simulink model "practica5_simulink"  (R2024a)
settings: Solver=ode4  StartTime=0.0  StopTime=0.5  FixedStep=0.000001  RelTol=1e-3
values from neighbouring files (symbols this model uses):
  den = [1, R/L, 1/(L*C)]    [pr5pt1.m]
  Kd = 0.01    [pr5pt1.m]
  Ki = 1000    [pr5pt1.m]
  Kp = 10    [pr5pt1.m]
  num = [1/(L*C)]    [pr5pt1.m]
libraries: slpidlib x3
settings Model: Creator=Monsty  LastModifiedBy=Monsty

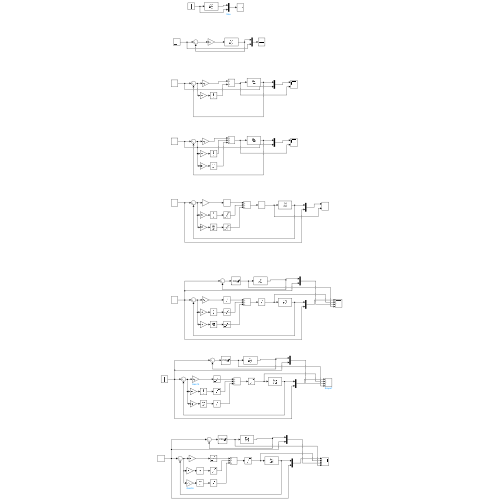
[thumbnail: Simulink's stored preview of the top-level diagram]
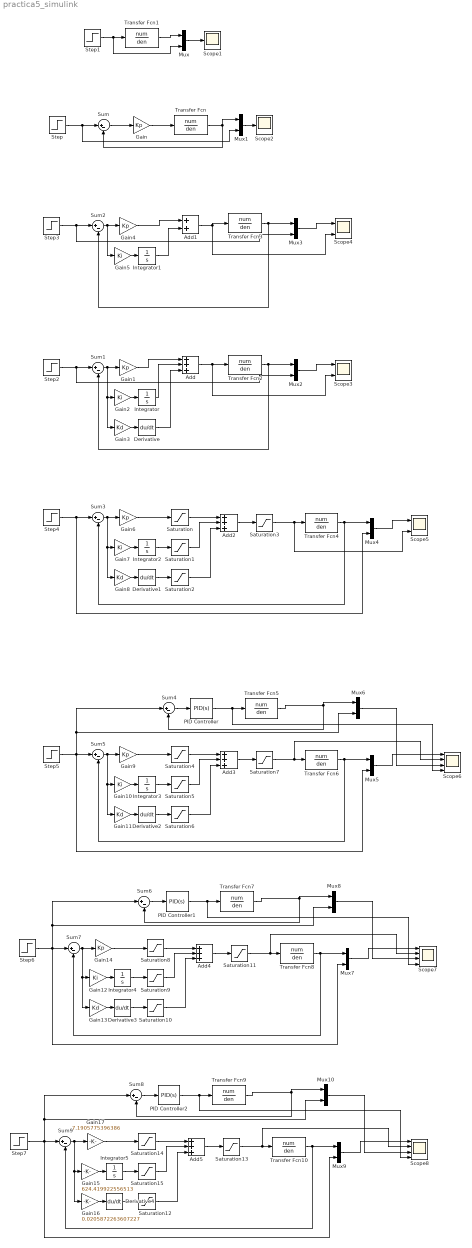
== system practica5_simulink ==
  Add{,2..5} (5 alike) : Sum  Inputs=+++
  Add1 : Sum
  Derivative{,1..4} (5 alike) : Derivative
  Gain{,1,4,6,9,14} (6 alike) : Gain  Gain=Kp
  Gain{2,5,7,10,12} (5 alike) : Gain  Gain=Ki
  Gain{3,8,11,13} (4 alike) : Gain  Gain=Kd
  Gain15 : Gain  Gain=624.419922556513
  Gain16 : Gain  Gain=0.0205872263607227
  Gain17 : Gain  Gain=7.1905775396386
  Integrator{,1..5} (6 alike) : Integrator
  Mux{,1..10} (11 alike) : Mux  Inputs=2
  PID Controller : slpidlib/PID Controller  Controller=PID  Form=Parallel  TimeDomain=Continuous-time  UseExternalTs=off  SampleTime=-1  IntegratorMethod=Forward Euler  FilterMethod=Forward Euler  ControllerParametersSource=internal  P=10  I=100  UseKiTs=off  D=0.01  UseExternalDerivativeSource=off  N=1000000  UseFilter=on  TunerSelectOption=Transfer Function Based (PID Tuner App)  InitialConditionSource=internal  InitialConditionForIntegrator=0  InitialConditionForFilter=0  DifferentiatorICPrevScaledInput=0  ExternalReset=none  TrackingMode=off  Kt=1  LimitOutput=on  SatLimitsSource=internal  UpperSaturationLimit=15  LowerSaturationLimit=-15  LinearizeAsGain=on  AntiWindupMode=none  Kb=1  LimitIntegrator=off  UpperIntegratorSaturationLimit=inf  LowerIntegratorSaturationLimit=-inf  POutMin=[]  POutMax=[]  IOutMin=[]  IOutMax=[]  DOutMin=[]  DOutMax=[]  NOutMin=[]  NOutMax=[]  SumOutMin=[]  SumOutMax=[]  SaturationOutMin=[]  SaturationOutMax=[]  PParamMin=[]  PParamMax=[]  IParamMin=[]  IParamMax=[]  DParamMin=[]  DParamMax=[]  NParamMin=[]  NParamMax=[]  KbParamMin=[]  KbParamMax=[]  KtParamMin=[]  KtParamMax=[]  KbOutMin=[]  KbOutMax=[]  KtOutMin=[]  KtOutMax=[]  IntegratorOutMin=[]  IntegratorOutMax=[]  FilterOutMin=[]  FilterOutMax=[]  SumI1OutMin=[]  SumI1OutMax=[]  SumI2OutMin=[]  SumI2OutMax=[]  SumI3OutMin=[]  SumI3OutMax=[]  SumI4OutMin=[]  SumI4OutMax=[]  SumDOutMin=[]  SumDOutMax=[]  DifferentiatorOutMin=[]  DifferentiatorOutMax=[]  FilterDiffOutCoefMin=[]  FilterDiffOutCoefMax=[]  ReciprocalOutMin=[]  ReciprocalOutMax=[]  SumDenOutMin=[]  SumDenOutMax=[]  SumNumOutMin=[]  SumNumOutMax=[]  DivideOutMin=[]  DivideOutMax=[]  UdiffTsProdOutMin=[]  UdiffTsProdOutMax=[]  NTsProdOutMin=[]  NTsProdOutMax=[]  UintegralTsProdOutMin=[]  UintegralTsProdOutMax=[]  UngainTsProdOutMin=[]  UngainTsProdOutMax=[]  ClampingZeroOutDataTypeStr=Inherit: Inherit via back propagation  ClampingZeroOutMin=[]  ClampingZeroOutMax=[]  FilterDenConstantOutDataTypeStr=Inherit: Inherit via back propagation  FilterDenConstantOutMin=[]  FilterDenConstantOutMax=[]  PCopyOutDataTypeStr=Inherit: Inherit via back propagation  PCopyOutMin=[]  PCopyOutMax=[]  NCopyOutDataTypeStr=Inherit: Inherit via back propagation  NCopyOutMin=[]  NCopyOutMax=[]  IntegratorContinuousStateAttributes=''  IntegratorStateMustResolveToSignalObject=off  IntegratorRTWStateStorageClass=Auto  FilterContinuousStateAttributes=''  FilterStateMustResolveToSignalObject=off  FilterRTWStateStorageClass=Auto  ParallelPVariant=InternalParameters  IdealPVariant=Disabled  IVariant=InternalParameters  DVariant=InternalParameters  IntegratorVariant=Continuous  SatVariant=Enabled  AWVariant=Passthrough  PCopyVariant=Disabled  TRVariant=Disabled  FdbkBlocksVariant=Forward  IdealPFdbkVariant=Disabled  SatFdbkVariant=Disabled  DerivativeFilterVariant=ContFilter  NVariant=InternalParameters  NCopyVariant=Disabled  FilterICVariant=InternalICsFilter  IntegratorICVariant=InternalICs  ExternalResetVariant=Disabled  TRSumVariant=Passthrough  SumFdbkVariant=Disabled  SumVariant=Sum_PID  TsampFilterVariant=InternalTs  TsampNgainVariant=Passthrough  TsampIntegralVariant=Disabled_SignalSpec  ExternalSaturationOutDataTypeStr=Inherit: Same as second input  DerivativeSourceVariant=ErrorSignal
  PID Controller1 : slpidlib/PID Controller  Controller=PID  Form=Parallel  TimeDomain=Continuous-time  UseExternalTs=off  SampleTime=-1  IntegratorMethod=Forward Euler  FilterMethod=Forward Euler  ControllerParametersSource=internal  P=7.1905775396386  I=624.419922556513  UseKiTs=off  D=0.0205872263607227  UseExternalDerivativeSource=off  N=115459.593100322  UseFilter=on  TunerSelectOption=Transfer Function Based (PID Tuner App)  InitialConditionSource=internal  InitialConditionForIntegrator=0  InitialConditionForFilter=0  DifferentiatorICPrevScaledInput=0  ExternalReset=none  TrackingMode=off  Kt=1  LimitOutput=on  SatLimitsSource=internal  UpperSaturationLimit=15  LowerSaturationLimit=-15  LinearizeAsGain=on  AntiWindupMode=none  Kb=1  LimitIntegrator=off  UpperIntegratorSaturationLimit=inf  LowerIntegratorSaturationLimit=-inf  POutMin=[]  POutMax=[]  IOutMin=[]  IOutMax=[]  DOutMin=[]  DOutMax=[]  NOutMin=[]  NOutMax=[]  SumOutMin=[]  SumOutMax=[]  SaturationOutMin=[]  SaturationOutMax=[]  PParamMin=[]  PParamMax=[]  IParamMin=[]  IParamMax=[]  DParamMin=[]  DParamMax=[]  NParamMin=[]  NParamMax=[]  KbParamMin=[]  KbParamMax=[]  KtParamMin=[]  KtParamMax=[]  KbOutMin=[]  KbOutMax=[]  KtOutMin=[]  KtOutMax=[]  IntegratorOutMin=[]  IntegratorOutMax=[]  FilterOutMin=[]  FilterOutMax=[]  SumI1OutMin=[]  SumI1OutMax=[]  SumI2OutMin=[]  SumI2OutMax=[]  SumI3OutMin=[]  SumI3OutMax=[]  SumI4OutMin=[]  SumI4OutMax=[]  SumDOutMin=[]  SumDOutMax=[]  DifferentiatorOutMin=[]  DifferentiatorOutMax=[]  FilterDiffOutCoefMin=[]  FilterDiffOutCoefMax=[]  ReciprocalOutMin=[]  ReciprocalOutMax=[]  SumDenOutMin=[]  SumDenOutMax=[]  SumNumOutMin=[]  SumNumOutMax=[]  DivideOutMin=[]  DivideOutMax=[]  UdiffTsProdOutMin=[]  UdiffTsProdOutMax=[]  NTsProdOutMin=[]  NTsProdOutMax=[]  UintegralTsProdOutMin=[]  UintegralTsProdOutMax=[]  UngainTsProdOutMin=[]  UngainTsProdOutMax=[]  ClampingZeroOutDataTypeStr=Inherit: Inherit via back propagation  ClampingZeroOutMin=[]  ClampingZeroOutMax=[]  FilterDenConstantOutDataTypeStr=Inherit: Inherit via back propagation  FilterDenConstantOutMin=[]  FilterDenConstantOutMax=[]  PCopyOutDataTypeStr=Inherit: Inherit via back propagation  PCopyOutMin=[]  PCopyOutMax=[]  NCopyOutDataTypeStr=Inherit: Inherit via back propagation  NCopyOutMin=[]  NCopyOutMax=[]  IntegratorContinuousStateAttributes=''  IntegratorStateMustResolveToSignalObject=off  IntegratorRTWStateStorageClass=Auto  FilterContinuousStateAttributes=''  FilterStateMustResolveToSignalObject=off  FilterRTWStateStorageClass=Auto  ParallelPVariant=InternalParameters  IdealPVariant=Disabled  IVariant=InternalParameters  DVariant=InternalParameters  IntegratorVariant=Continuous  SatVariant=Enabled  AWVariant=Passthrough  PCopyVariant=Disabled  TRVariant=Disabled  FdbkBlocksVariant=Forward  IdealPFdbkVariant=Disabled  SatFdbkVariant=Disabled  DerivativeFilterVariant=ContFilter  NVariant=InternalParameters  NCopyVariant=Disabled  FilterICVariant=InternalICsFilter  IntegratorICVariant=InternalICs  ExternalResetVariant=Disabled  TRSumVariant=Passthrough  SumFdbkVariant=Disabled  SumVariant=Sum_PID  TsampFilterVariant=InternalTs  TsampNgainVariant=Passthrough  TsampIntegralVariant=Disabled_SignalSpec  ExternalSaturationOutDataTypeStr=Inherit: Same as second input  DerivativeSourceVariant=ErrorSignal
  PID Controller2 : slpidlib/PID Controller  Controller=PID  Form=Parallel  TimeDomain=Continuous-time  UseExternalTs=off  SampleTime=-1  IntegratorMethod=Forward Euler  FilterMethod=Forward Euler  ControllerParametersSource=internal  P=7.1905775396386  I=624.419922556513  UseKiTs=off  D=0.0205872263607227  UseExternalDerivativeSource=off  N=115459.593100322  UseFilter=on  TunerSelectOption=Transfer Function Based (PID Tuner App)  InitialConditionSource=internal  InitialConditionForIntegrator=0  InitialConditionForFilter=0  DifferentiatorICPrevScaledInput=0  ExternalReset=none  TrackingMode=off  Kt=1  LimitOutput=on  SatLimitsSource=internal  UpperSaturationLimit=15  LowerSaturationLimit=-15  LinearizeAsGain=on  AntiWindupMode=none  Kb=1  LimitIntegrator=off  UpperIntegratorSaturationLimit=inf  LowerIntegratorSaturationLimit=-inf  POutMin=[]  POutMax=[]  IOutMin=[]  IOutMax=[]  DOutMin=[]  DOutMax=[]  NOutMin=[]  NOutMax=[]  SumOutMin=[]  SumOutMax=[]  SaturationOutMin=[]  SaturationOutMax=[]  PParamMin=[]  PParamMax=[]  IParamMin=[]  IParamMax=[]  DParamMin=[]  DParamMax=[]  NParamMin=[]  NParamMax=[]  KbParamMin=[]  KbParamMax=[]  KtParamMin=[]  KtParamMax=[]  KbOutMin=[]  KbOutMax=[]  KtOutMin=[]  KtOutMax=[]  IntegratorOutMin=[]  IntegratorOutMax=[]  FilterOutMin=[]  FilterOutMax=[]  SumI1OutMin=[]  SumI1OutMax=[]  SumI2OutMin=[]  SumI2OutMax=[]  SumI3OutMin=[]  SumI3OutMax=[]  SumI4OutMin=[]  SumI4OutMax=[]  SumDOutMin=[]  SumDOutMax=[]  DifferentiatorOutMin=[]  DifferentiatorOutMax=[]  FilterDiffOutCoefMin=[]  FilterDiffOutCoefMax=[]  ReciprocalOutMin=[]  ReciprocalOutMax=[]  SumDenOutMin=[]  SumDenOutMax=[]  SumNumOutMin=[]  SumNumOutMax=[]  DivideOutMin=[]  DivideOutMax=[]  UdiffTsProdOutMin=[]  UdiffTsProdOutMax=[]  NTsProdOutMin=[]  NTsProdOutMax=[]  UintegralTsProdOutMin=[]  UintegralTsProdOutMax=[]  UngainTsProdOutMin=[]  UngainTsProdOutMax=[]  ClampingZeroOutDataTypeStr=Inherit: Inherit via back propagation  ClampingZeroOutMin=[]  ClampingZeroOutMax=[]  FilterDenConstantOutDataTypeStr=Inherit: Inherit via back propagation  FilterDenConstantOutMin=[]  FilterDenConstantOutMax=[]  PCopyOutDataTypeStr=Inherit: Inherit via back propagation  PCopyOutMin=[]  PCopyOutMax=[]  NCopyOutDataTypeStr=Inherit: Inherit via back propagation  NCopyOutMin=[]  NCopyOutMax=[]  IntegratorContinuousStateAttributes=''  IntegratorStateMustResolveToSignalObject=off  IntegratorRTWStateStorageClass=Auto  FilterContinuousStateAttributes=''  FilterStateMustResolveToSignalObject=off  FilterRTWStateStorageClass=Auto  ParallelPVariant=InternalParameters  IdealPVariant=Disabled  IVariant=InternalParameters  DVariant=InternalParameters  IntegratorVariant=Continuous  SatVariant=Enabled  AWVariant=Passthrough  PCopyVariant=Disabled  TRVariant=Disabled  FdbkBlocksVariant=Forward  IdealPFdbkVariant=Disabled  SatFdbkVariant=Disabled  DerivativeFilterVariant=ContFilter  NVariant=InternalParameters  NCopyVariant=Disabled  FilterICVariant=InternalICsFilter  IntegratorICVariant=InternalICs  ExternalResetVariant=Disabled  TRSumVariant=Passthrough  SumFdbkVariant=Disabled  SumVariant=Sum_PID  TsampFilterVariant=InternalTs  TsampNgainVariant=Passthrough  TsampIntegralVariant=Disabled_SignalSpec  ExternalSaturationOutDataTypeStr=Inherit: Same as second input  DerivativeSourceVariant=ErrorSignal
  Saturation{,1..15} (16 alike) : Saturate  UpperLimit=15  LowerLimit=-15
  Scope1 : Scope
  Scope2 : Scope
  Scope3 : Scope  NumInputPorts=2
  Scope4 : Scope  NumInputPorts=2
  Scope5 : Scope  NumInputPorts=2
  Scope6 : Scope  NumInputPorts=4
  Scope7 : Scope  NumInputPorts=4
  Scope8 : Scope  NumInputPorts=4
  Step{,1..3} (4 alike) : Step  Time=0.01  After=5  SampleTime=0
  Step{4..7} (4 alike) : Step  Time=0.05  SampleTime=0
  Sum{,1..9} (10 alike) : Sum  Inputs=|+-
  Transfer Fcn{,1..10} (11 alike) : TransferFcn  Numerator=num  Denominator=den
  wires:
  Sum/1 -> Gain/1
  Gain/1 -> Transfer Fcn/1
  Transfer Fcn/1 -> Mux1/1, Sum/2
  Mux/1 -> Scope1/1
  Transfer Fcn1/1 -> Mux/1
  Step1/1 -> Mux/2, Transfer Fcn1/1
  Step/1 -> Mux1/2, Sum/1
  Mux1/1 -> Scope2/1
  Step2/1 -> Mux2/2, Sum1/1
  Transfer Fcn2/1 -> Sum1/2, Mux2/1
  Sum1/1 -> Gain3/1, Gain2/1, Gain1/1
  Gain2/1 -> Integrator/1
  Add/1 -> Scope3/2, Transfer Fcn2/1
  Gain1/1 -> Add/1
  Integrator/1 -> Add/2
  Mux2/1 -> Scope3/1
  Gain3/1 -> Derivative/1
  Derivative/1 -> Add/3
  Sum2/1 -> Gain5/1, Gain4/1
  Step3/1 -> Mux3/2, Sum2/1
  Transfer Fcn3/1 -> Sum2/2, Mux3/1
  Integrator1/1 -> Add1/2
  Add1/1 -> Transfer Fcn3/1, Scope4/2
  Gain4/1 -> Add1/1
  Gain5/1 -> Integrator1/1
  Mux3/1 -> Scope4/1
  Sum3/1 -> Gain8/1, Gain7/1, Gain6/1
  Step4/1 -> Mux4/2, Sum3/1
  Transfer Fcn4/1 -> Mux4/1, Sum3/2
  Gain8/1 -> Derivative1/1
  Integrator2/1 -> Saturation1/1
  Derivative1/1 -> Saturation2/1
  Add2/1 -> Saturation3/1
  Gain6/1 -> Saturation/1
  Gain7/1 -> Integrator2/1
  Mux4/1 -> Scope5/1
  Saturation/1 -> Add2/1
  Saturation1/1 -> Add2/2
  Saturation2/1 -> Add2/3
  Saturation3/1 -> Transfer Fcn4/1, Scope5/2
  Sum4/1 -> PID Controller/1
  PID Controller/1 -> Scope6/4, Transfer Fcn5/1
  Saturation5/1 -> Add3/2
  Gain10/1 -> Integrator3/1
  Gain9/1 -> Saturation4/1
  Transfer Fcn6/1 -> Mux5/1, Sum5/2
  Derivative2/1 -> Saturation6/1
  Mux5/1 -> Scope6/1
  Gain11/1 -> Derivative2/1
  Integrator3/1 -> Saturation5/1
  Saturation6/1 -> Add3/3
  Sum5/1 -> Gain11/1, Gain10/1, Gain9/1
  Add3/1 -> Saturation7/1
  Saturation7/1 -> Transfer Fcn6/1, Scope6/2
  Saturation4/1 -> Add3/1
  Step5/1 -> Sum4/1, Mux6/2, Mux5/2, Sum5/1
  Transfer Fcn5/1 -> Sum4/2, Mux6/1
  Mux6/1 -> Scope6/3
  Transfer Fcn7/1 -> Sum6/2, Mux8/1
  PID Controller1/1 -> Scope7/4, Transfer Fcn7/1
  Mux8/1 -> Scope7/3
  Transfer Fcn8/1 -> Mux7/1, Sum7/2
  Saturation8/1 -> Add4/1
  Saturation10/1 -> Add4/3
  Saturation11/1 -> Transfer Fcn8/1, Scope7/2
  Sum7/1 -> Gain13/1, Gain12/1, Gain14/1
  Step6/1 -> Sum6/1, Mux8/2, Mux7/2, Sum7/1
  Add4/1 -> Saturation11/1
  Gain12/1 -> Integrator4/1
  Derivative3/1 -> Saturation10/1
  Gain13/1 -> Derivative3/1
  Gain14/1 -> Saturation8/1
  Mux7/1 -> Scope7/1
  Integrator4/1 -> Saturation9/1
  Saturation9/1 -> Add4/2
  Sum6/1 -> PID Controller1/1
  Step7/1 -> Sum8/1, Mux10/2, Mux9/2, Sum9/1
  Gain15/1 -> Integrator5/1
  Add5/1 -> Saturation13/1
  Mux10/1 -> Scope8/3
  Saturation14/1 -> Add5/1
  PID Controller2/1 -> Scope8/4, Transfer Fcn9/1
  Transfer Fcn9/1 -> Sum8/2, Mux10/1
  Sum9/1 -> Gain16/1, Gain15/1, Gain17/1
  Transfer Fcn10/1 -> Mux9/1, Sum9/2
  Saturation13/1 -> Transfer Fcn10/1, Scope8/2
  Derivative4/1 -> Saturation12/1
  Mux9/1 -> Scope8/1
  Gain17/1 -> Saturation14/1
  Saturation15/1 -> Add5/2
  Sum8/1 -> PID Controller2/1
  Gain16/1 -> Derivative4/1
  Integrator5/1 -> Saturation15/1
  Saturation12/1 -> Add5/3
